simulink model "ThreeSpeciesModel"  (R2024b)
settings: Solver=FixedStepDiscrete  StartTime=0.0  StopTime=10.0  FixedStep=0.001  RelTol=1e-3
undefined symbols (not defined in the file): b0, CC1, CC2, k1, k2, n, p0, s0, x
settings Model: Creator=JTerr  LastModifiedBy=JTerr

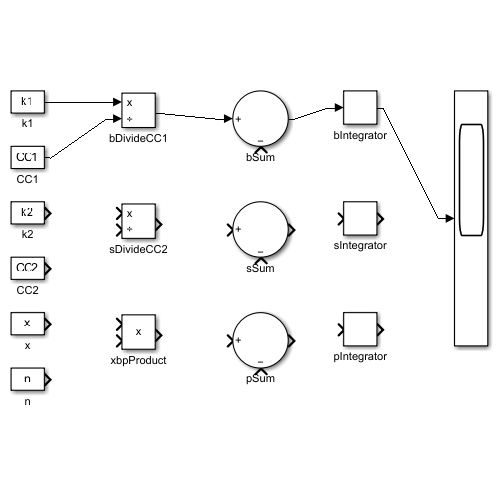
[thumbnail: Simulink's stored preview of the top-level diagram]
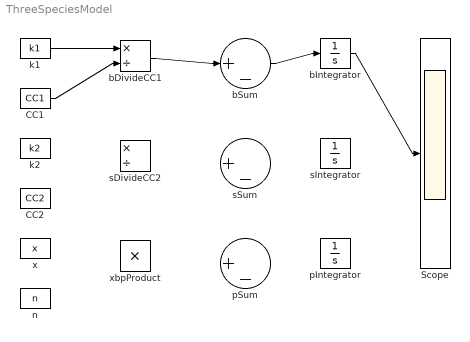
== system ThreeSpeciesModel ==
  CC1 : Constant  Value=CC1
  CC2 : Constant  Value=CC2
  Scope : Scope
  bDivideCC1 : Product  Inputs=*/
  bIntegrator : Integrator  InitialCondition=b0
  bSum : Sum  Inputs=|+-
  k1 : Constant  Value=k1
  k2 : Constant  Value=k2
  n : Constant  Value=n
  pIntegrator : Integrator  InitialCondition=p0
  pSum : Sum  Inputs=|+-
  sDivideCC2 : Product  Inputs=*/
  sIntegrator : Integrator  InitialCondition=s0
  sSum : Sum  Inputs=|+-
  x : Constant  Value=x
  xbpProduct : Product
  wires:
  k1/1 -> bDivideCC1/1
  CC1/1 -> bDivideCC1/2
  bDivideCC1/1 -> bSum/1
  bSum/1 -> bIntegrator/1
  bIntegrator/1 -> Scope/1
